simulink model "aux"  (R2018b)
settings: Solver=VariableStepAuto  StartTime=0.0  StopTime=1000  RelTol=1e-3
values from neighbouring files (symbols this model uses):
  y0 = [x0;x_hat_0;theta_star_0]    [aux.m]
undefined symbols (not defined in the file or in its folder): alphaInstant, alphaIntegral, alphaLeastSquares, beta0, betaIntegral, betaLeast, GammaInstant, GammaIntegral, k0, lambda1, lambda2, m0, P0, R0, rho0, rho1, taskE, theta0, y_dot0
libraries: dspmtrx3 x1
settings Model: Creator=cale  LastModifiedBy=cale

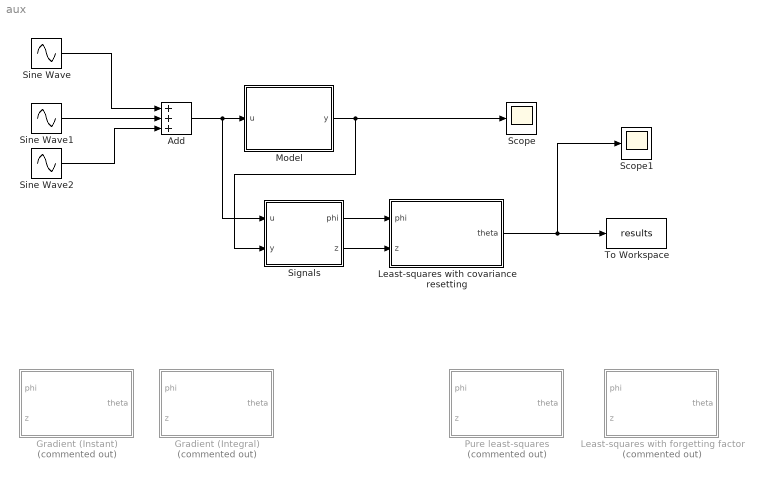
== system aux ==
  Add : Sum  Inputs=3
  Gradient (Instant) : Subsystem  Commented=on
  Gradient (Integral) : Subsystem  Commented=on
  Least-squares with covariance resetting : Subsystem
  Least-squares with forgetting factor : Subsystem  Commented=on
  Model : Subsystem
  Pure least-squares : Subsystem  Commented=on
  Scope : Scope
  Scope1 : Scope
  Signals : Subsystem
  Sine Wave : Sin  Amplitude=3  Frequency=0.1  SampleTime=0
  Sine Wave1 : Sin  Frequency=5  SampleTime=0
  Sine Wave2 : Sin  Amplitude=10  Frequency=3  SampleTime=0
  To Workspace : ToWorkspace  VariableName=results  SaveFormat=Timeseries  SampleTime=-1
  wires:
  Add/1 -> Signals/1("u "), Model/1(u)
  Model/1(y) -> Signals/2("y "), Scope/1
  Signals/1(phi) -> Least-squares with covariance resetting/1(phi)
  Least-squares with covariance resetting/1(theta) -> Scope1/1, To Workspace/1
  Sine Wave1/1 -> Add/2
  Sine Wave/1 -> Add/1
  Sine Wave2/1 -> Add/3
  Signals/2(z) -> Least-squares with covariance resetting/2(z)

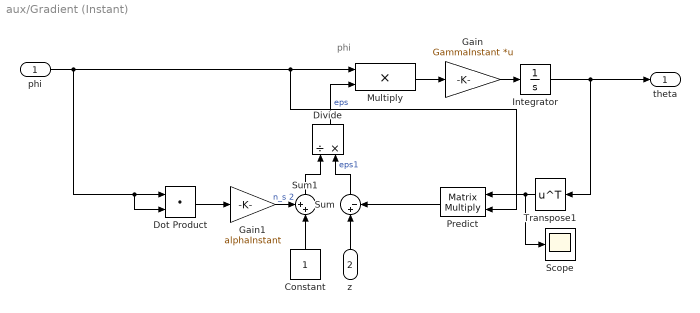
== system aux/Gradient (Instant) ==
  note: phi
  phi : Inport
  z : Inport  Port=2
  Constant : Constant
  Divide : Product  Inputs=/*
  Dot Product : DotProduct  InputSameDT=on  OutDataTypeStr=Inherit: Inherit via internal rule
  Gain : Gain  Gain=GammaInstant  Multiplication=Matrix(K*u) (u vector)
  Gain1 : Gain  Gain=alphaInstant
  Integrator : Integrator  InitialCondition=theta0
  Multiply : Product
  Predict : Product  Multiplication=Matrix(*)
  Scope : Scope
  Sum : Sum  Inputs=|+-
  Sum1 : Sum  Inputs=++|
  Transpose1 : Math  Operator=transpose  SaturateOnIntegerOverflow=on
  theta : Outport
  wires:
  Multiply/1 -> Gain/1
  Gain/1 -> Integrator/1
  z/1 -> Sum/1
  Predict/1 -> Sum/2
  Sum/1 -> Divide/2  "eps1"
  Gain1/1 -> Sum1/1  "n_s 2"
  Sum1/1 -> Divide/1
  Constant/1 -> Sum1/2
  Divide/1 -> Multiply/2  "eps"
  Integrator/1 -> Transpose1/1, theta/1
  phi/1 -> Dot Product/2, Dot Product/1, Predict/2, Multiply/1
  Transpose1/1 -> Scope/1, Predict/1
  Dot Product/1 -> Gain1/1

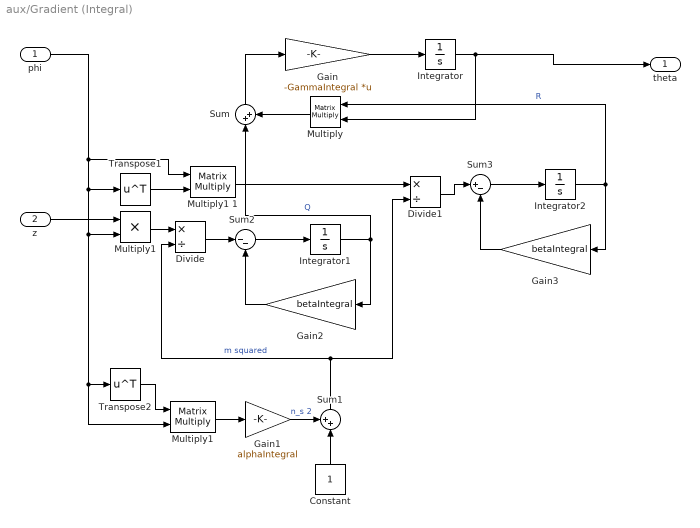
== system aux/Gradient (Integral) ==
  phi : Inport
  z : Inport  Port=2
  Constant : Constant
  Divide : Product  Inputs=*/
  Divide1 : Product  Inputs=*/
  Gain : Gain  Gain=-GammaIntegral  Multiplication=Matrix(K*u) (u vector)
  Gain1 : Gain  Gain=alphaIntegral
  Gain2 : Gain  Gain=betaIntegral
  Gain3 : Gain  Gain=betaIntegral
  Integrator : Integrator  InitialCondition=theta0
  Integrator1 : Integrator
  Integrator2 : Integrator
  Multiply : Product  Multiplication=Matrix(*)
  Multiply1 : Product
  "Multiply1 " : Product  Multiplication=Matrix(*)
  Multiply1 1 : Product  Multiplication=Matrix(*)
  Sum : Sum  Inputs=|++
  Sum1 : Sum  Inputs=++|
  Sum2 : Sum  Inputs=|--
  Sum3 : Sum  Inputs=|+-
  Transpose1 : Math  Operator=transpose  SaturateOnIntegerOverflow=on
  Transpose2 : Math  Operator=transpose  SaturateOnIntegerOverflow=on
  theta : Outport
  wires:
  Gain/1 -> Integrator/1
  Gain1/1 -> Sum1/1  "n_s 2"
  Sum1/1 -> Divide/2, Divide1/2  "m squared"
  Constant/1 -> Sum1/2
  Integrator/1 -> Multiply/2, theta/1
  Transpose2/1 -> "Multiply1 "/1
  "Multiply1 "/1 -> Gain1/1
  Integrator1/1 -> Gain2/1, Sum/1  "Q"
  Sum2/1 -> Integrator1/1
  Gain2/1 -> Sum2/2
  z/1 -> Multiply1/1
  Divide/1 -> Sum2/1
  Multiply1/1 -> Divide/1
  Integrator2/1 -> Multiply/1, Gain3/1  "R"
  Gain3/1 -> Sum3/2
  Sum3/1 -> Integrator2/1
  Divide1/1 -> Sum3/1
  Sum/1 -> Gain/1
  Multiply/1 -> Sum/2
  Transpose1/1 -> Multiply1 1/2
  phi/1 -> Transpose1/1, Multiply1/2, "Multiply1 "/2, Transpose2/1, Multiply1 1/1
  Multiply1 1/1 -> Divide1/1

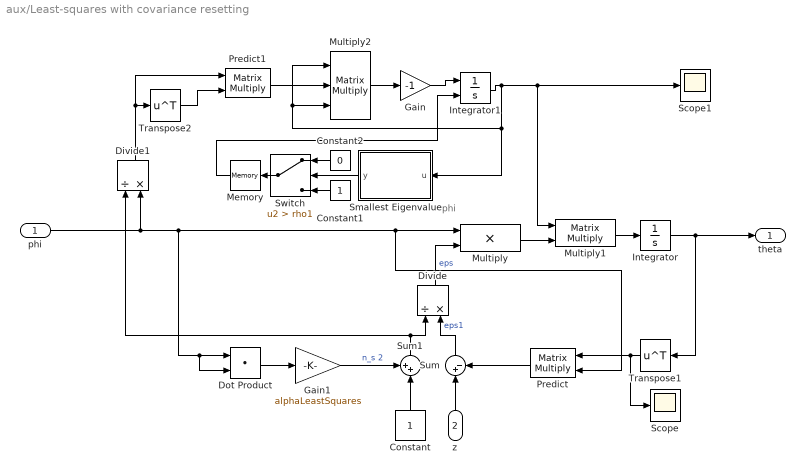
== system aux/Least-squares with covariance resetting ==
  note: phi
  phi : Inport
  z : Inport  Port=2
  Constant : Constant
  Constant1 : Constant
  Constant2 : Constant  Value=0
  Divide : Product  Inputs=/*
  Divide1 : Product  Inputs=/*
  Dot Product : DotProduct  InputSameDT=on  OutDataTypeStr=Inherit: Inherit via internal rule
  Gain : Gain  Gain=-1
  Gain1 : Gain  Gain=alphaLeastSquares
  Integrator : Integrator  InitialCondition=theta0
  Integrator1 : Integrator  ExternalReset=rising  InitialCondition=rho0*eye(3)
  Memory : Memory
  Multiply : Product
  Multiply1 : Product  Multiplication=Matrix(*)
  Multiply2 : Product  Inputs=3  Multiplication=Matrix(*)
  Predict : Product  Multiplication=Matrix(*)
  Predict1 : Product  Multiplication=Matrix(*)
  Scope : Scope
  Scope1 : Scope
  Smallest Eigenvalue : MATLAB Function  TreatAsAtomicUnit=on
  Sum : Sum  Inputs=|+-
  Sum1 : Sum  Inputs=++|
  Switch : Switch  Criteria=u2 > Threshold  Threshold=rho1
  Transpose1 : Math  Operator=transpose  SaturateOnIntegerOverflow=on
  Transpose2 : Math  Operator=transpose  SaturateOnIntegerOverflow=on
  theta : Outport
  wires:
  Multiply/1 -> Multiply1/2
  Multiply1/1 -> Integrator/1
  z/1 -> Sum/1
  Predict/1 -> Sum/2
  Sum/1 -> Divide/2  "eps1"
  Gain1/1 -> Sum1/1  "n_s 2"
  Sum1/1 -> Divide1/1, Divide/1
  Constant/1 -> Sum1/2
  Divide/1 -> Multiply/2  "eps"
  Integrator/1 -> Transpose1/1, theta/1
  phi/1 -> Dot Product/2, Dot Product/1, Predict/2, Multiply/1, Divide1/2
  Transpose1/1 -> Scope/1, Predict/1
  Dot Product/1 -> Gain1/1
  Multiply2/1 -> Gain/1
  Predict1/1 -> Multiply2/2
  Gain/1 -> Integrator1/1
  Transpose2/1 -> Predict1/2
  Divide1/1 -> Predict1/1, Transpose2/1
  Integrator1/1 -> Smallest Eigenvalue/1(u), Multiply2/3, Multiply2/1, Scope1/1, Multiply1/1
  Smallest Eigenvalue/1(y) -> Switch/2
  Constant1/1 -> Switch/3
  Switch/1 -> Memory/1
  Memory/1 -> Integrator1/2
  Constant2/1 -> Switch/1

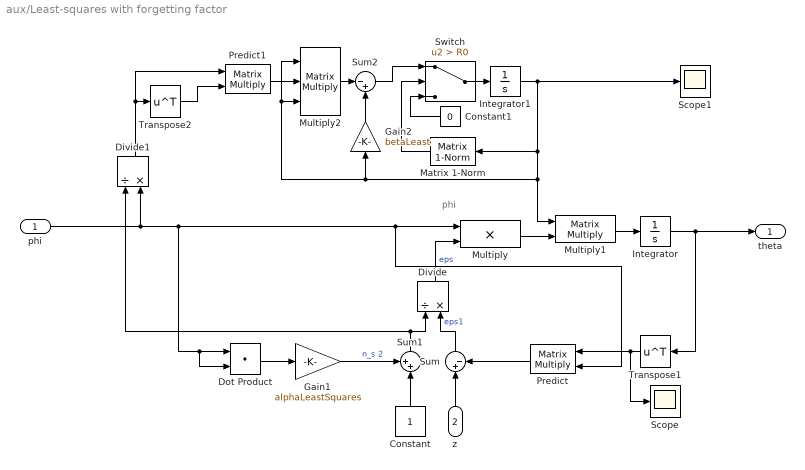
== system aux/Least-squares with forgetting factor ==
  note: phi
  phi : Inport
  z : Inport  Port=2
  Constant : Constant
  Constant1 : Constant  Value=0
  Divide : Product  Inputs=/*
  Divide1 : Product  Inputs=/*
  Dot Product : DotProduct  InputSameDT=on  OutDataTypeStr=Inherit: Inherit via internal rule
  Gain1 : Gain  Gain=alphaLeastSquares
  Gain2 : Gain  Gain=betaLeast
  Integrator : Integrator  InitialCondition=theta0
  Integrator1 : Integrator  InitialCondition=P0
  Matrix 1-Norm : dspmtrx3/Matrix  1-Norm  roundingMode=Floor  overflowMode=off  outputDataTypeStr=Inherit: Same as accumulator  outputMin=[]  outputMax=[]  outputLastDataTypeStr=Inherit: Same as accumulator
      settings: SourceProductName=DSP System Toolbox  SourceProductBaseCode=DS
  Multiply : Product
  Multiply1 : Product  Multiplication=Matrix(*)
  Multiply2 : Product  Inputs=3  Multiplication=Matrix(*)
  Predict : Product  Multiplication=Matrix(*)
  Predict1 : Product  Multiplication=Matrix(*)
  Scope : Scope
  Scope1 : Scope
  Sum : Sum  Inputs=|+-
  Sum1 : Sum  Inputs=++|
  Sum2 : Sum  Inputs=|-+
  Switch : Switch  Criteria=u2 > Threshold  Threshold=R0
  Transpose1 : Math  Operator=transpose  SaturateOnIntegerOverflow=on
  Transpose2 : Math  Operator=transpose  SaturateOnIntegerOverflow=on
  theta : Outport
  wires:
  Multiply/1 -> Multiply1/2
  Multiply1/1 -> Integrator/1
  z/1 -> Sum/1
  Predict/1 -> Sum/2
  Sum/1 -> Divide/2  "eps1"
  Gain1/1 -> Sum1/1  "n_s 2"
  Sum1/1 -> Divide1/1, Divide/1
  Constant/1 -> Sum1/2
  Divide/1 -> Multiply/2  "eps"
  Integrator/1 -> Transpose1/1, theta/1
  phi/1 -> Dot Product/2, Dot Product/1, Predict/2, Multiply/1, Divide1/2
  Transpose1/1 -> Scope/1, Predict/1
  Dot Product/1 -> Gain1/1
  Predict1/1 -> Multiply2/2
  Transpose2/1 -> Predict1/2
  Divide1/1 -> Predict1/1, Transpose2/1
  Integrator1/1 -> Matrix 1-Norm/1, Gain2/1, Multiply2/3, Multiply2/1, Multiply1/1, Scope1/1
  Multiply2/1 -> Sum2/1
  Gain2/1 -> Sum2/2
  Switch/1 -> Integrator1/1
  Sum2/1 -> Switch/1
  Constant1/1 -> Switch/3
  Matrix 1-Norm/1 -> Switch/2

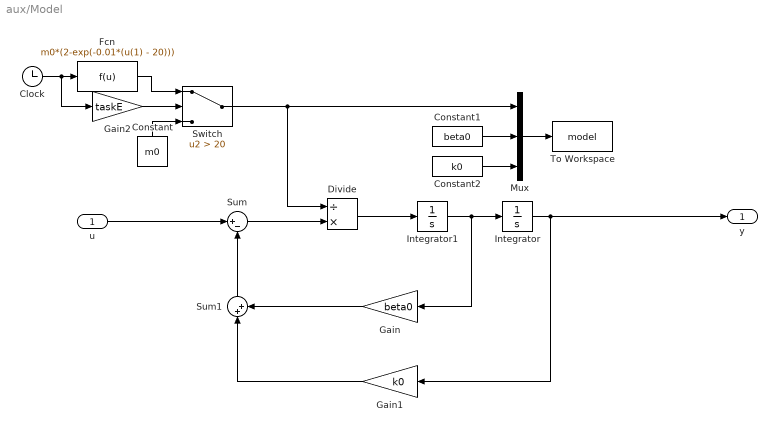
== system aux/Model ==
  u : Inport
  Clock : Clock
  Constant : Constant  Value=m0
  Constant1 : Constant  Value=beta0
  Constant2 : Constant  Value=k0
  Divide : Product  Inputs=/*
  Fcn : Fcn  Expr=m0*(2-exp(-0.01*(u(1) - 20)))
  Gain : Gain  Gain=beta0
  Gain1 : Gain  Gain=k0
  Gain2 : Gain  Gain=taskE
  Integrator : Integrator  InitialCondition=y0
  Integrator1 : Integrator  InitialCondition=y_dot0
  Mux : Mux  Inputs=3
  Sum : Sum  Inputs=|+-
  Sum1 : Sum  Inputs=|++
  Switch : Switch  Criteria=u2 > Threshold  Threshold=20
  To Workspace : ToWorkspace  VariableName=model  SaveFormat=Timeseries  SampleTime=-1
  y : Outport
  wires:
  Gain1/1 -> Sum1/1
  Sum/1 -> Divide/2
  u/1 -> Sum/1
  Sum1/1 -> Sum/2
  Gain/1 -> Sum1/2
  Integrator/1 -> y/1, Gain1/1
  Divide/1 -> Integrator1/1
  Integrator1/1 -> Gain/1, Integrator/1
  Mux/1 -> To Workspace/1
  Constant1/1 -> Mux/2
  Constant2/1 -> Mux/3
  Switch/1 -> Mux/1, Divide/1
  Clock/1 -> Gain2/1, Fcn/1
  Fcn/1 -> Switch/1
  Constant/1 -> Switch/3
  Gain2/1 -> Switch/2

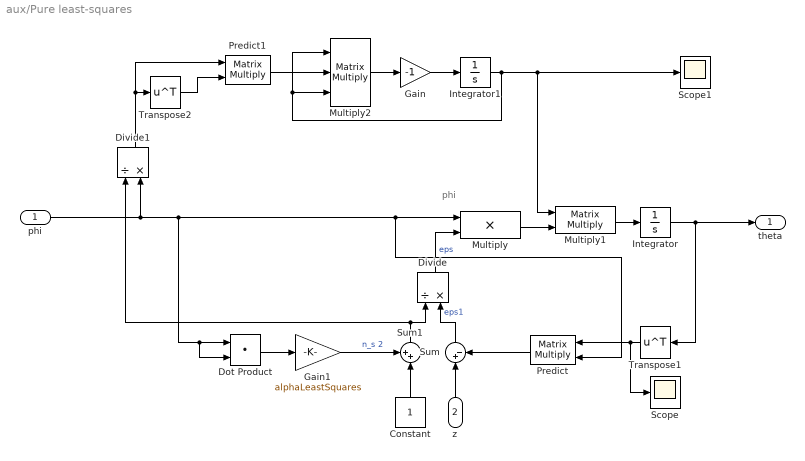
== system aux/Pure least-squares ==
  note: phi
  phi : Inport
  z : Inport  Port=2
  Constant : Constant
  Divide : Product  Inputs=/*
  Divide1 : Product  Inputs=/*
  Dot Product : DotProduct  InputSameDT=on  OutDataTypeStr=Inherit: Inherit via internal rule
  Gain : Gain  Gain=-1
  Gain1 : Gain  Gain=alphaLeastSquares
  Integrator : Integrator  InitialCondition=theta0
  Integrator1 : Integrator  InitialCondition=P0
  Multiply : Product
  Multiply1 : Product  Multiplication=Matrix(*)
  Multiply2 : Product  Inputs=3  Multiplication=Matrix(*)
  Predict : Product  Multiplication=Matrix(*)
  Predict1 : Product  Multiplication=Matrix(*)
  Scope : Scope
  Scope1 : Scope
  Sum : Sum  Inputs=|+-
  Sum1 : Sum  Inputs=++|
  Transpose1 : Math  Operator=transpose  SaturateOnIntegerOverflow=on
  Transpose2 : Math  Operator=transpose  SaturateOnIntegerOverflow=on
  theta : Outport
  wires:
  Multiply/1 -> Multiply1/2
  Multiply1/1 -> Integrator/1
  z/1 -> Sum/1
  Predict/1 -> Sum/2
  Sum/1 -> Divide/2  "eps1"
  Gain1/1 -> Sum1/1  "n_s 2"
  Sum1/1 -> Divide1/1, Divide/1
  Constant/1 -> Sum1/2
  Divide/1 -> Multiply/2  "eps"
  Integrator/1 -> Transpose1/1, theta/1
  phi/1 -> Dot Product/2, Dot Product/1, Predict/2, Multiply/1, Divide1/2
  Transpose1/1 -> Scope/1, Predict/1
  Dot Product/1 -> Gain1/1
  Multiply2/1 -> Gain/1
  Predict1/1 -> Multiply2/2
  Gain/1 -> Integrator1/1
  Transpose2/1 -> Predict1/2
  Divide1/1 -> Predict1/1, Transpose2/1
  Integrator1/1 -> Multiply2/3, Multiply2/1, Scope1/1, Multiply1/1

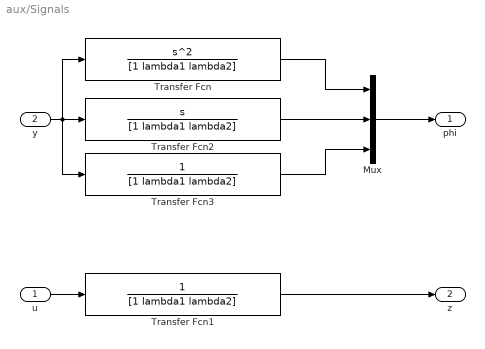
== system aux/Signals ==
  "u " : Inport
  "y " : Inport  Port=2
  Mux : Mux  Inputs=3
  Transfer Fcn : TransferFcn  Numerator=[1 0 0]  Denominator=[1 lambda1 lambda2]
  Transfer Fcn1 : TransferFcn  Denominator=[1 lambda1 lambda2]
  Transfer Fcn2 : TransferFcn  Numerator=[1 0]  Denominator=[1 lambda1 lambda2]
  Transfer Fcn3 : TransferFcn  Denominator=[1 lambda1 lambda2]
  phi : Outport
  z : Outport  Port=2
  wires:
  "y "/1 -> Transfer Fcn/1, Transfer Fcn3/1, Transfer Fcn2/1
  "u "/1 -> Transfer Fcn1/1
  Transfer Fcn1/1 -> z/1
  Mux/1 -> phi/1
  Transfer Fcn/1 -> Mux/1
  Transfer Fcn2/1 -> Mux/2
  Transfer Fcn3/1 -> Mux/3

== matlab function aux/Least-squares with covariance resetting/Smallest Eigenvalue ==
  data: u input; y output
function y = fcn(u)

y = min(real(eig(u)));
